simulink model "gm_HDLLDPCEncoder_vs"  (R2024a)
settings: Solver=FixedStepDiscrete  StartTime=0.0  StopTime=stopTime  RelTol=1e-3
values from neighbouring files (symbols this model uses):
  fs = 1    [testLDPCEncoder.m]
undefined symbols (not defined in the file or in its folder): clk, clk_enable, reset_x
libraries: whdlutilities x14, whdledac x6, simulink x5, dspsrcs4 x4, hdlsllib x1, vivadosimlib x1, HDL_ieee_8021513 x1
settings Model: Creator=cotti  LastModifiedBy=cotti
settings OptimizationCC: BlockReduction=off  ConditionallyExecuteInputs=off  DefaultParameterBehavior=Inlined  InheritOutputTypeSmallerThanSingle=on  ReuseModelBlockBuffer=off
settings DebuggingCC: AlgebraicLoopMsg=error  InheritedTsInSrcMsg=none  SingleTaskRateTransMsg=error  UnconnectedInputMsg=warning  UnconnectedOutputMsg=warning  UnconnectedLineMsg=warning
settings HardwareCC: ProdBitPerPointer=32  ProdBitPerSizeT=32  ProdBitPerPtrDiffT=32  ProdLargestAtomicFloat=None  ProdIntDivRoundTo=Undefined  ProdEndianess=Unspecified  ProdWordSize=32  ProdHWDeviceType=ASIC/FPGA->ASIC/FPGA  TargetBitPerLong=64  TargetBitPerPointer=64  TargetBitPerSizeT=64  TargetBitPerPtrDiffT=64  TargetLongLongMode=on  TargetIntDivRoundTo=Zero  TargetEndianess=LittleEndian  TargetWordSize=64  TargetHWDeviceType=Custom Processor->MATLAB Host Computer  ProdEqTarget=off
settings RTWCC: GPUComputeCapability=3.5

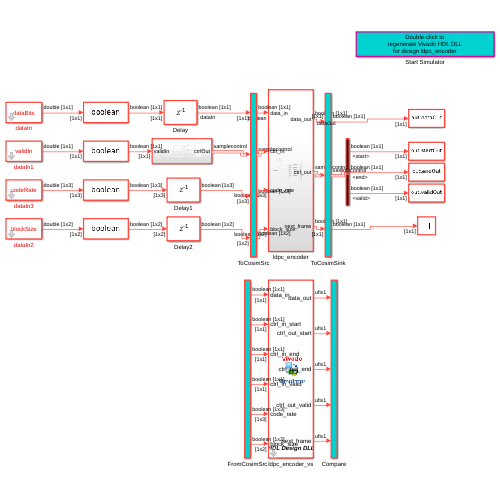
[thumbnail: Simulink's stored preview of the top-level diagram]
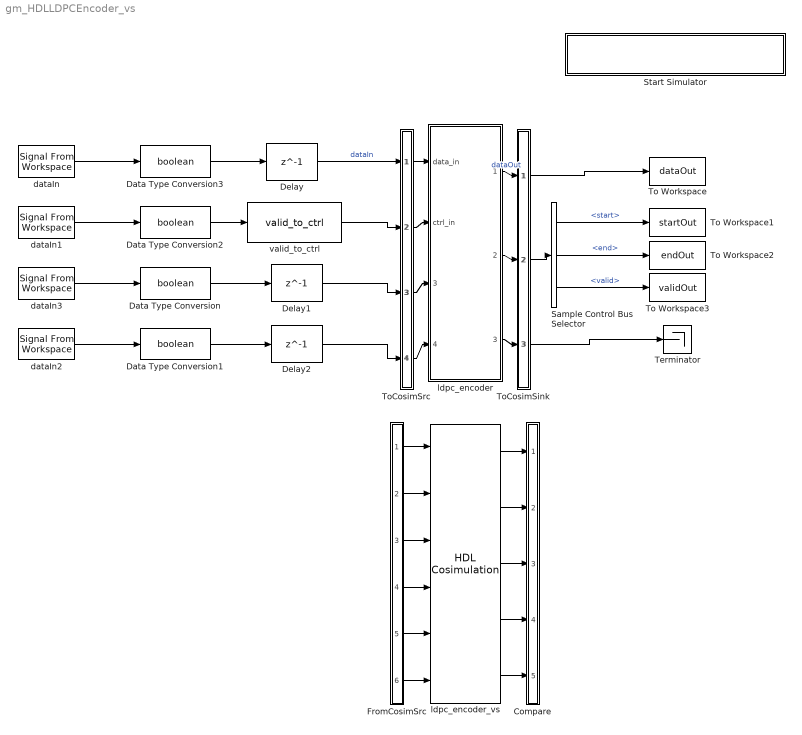
== system gm_HDLLDPCEncoder_vs ==
  Compare : Subsystem
      mask Display: disp('')
  Data Type Conversion{,1..3} (4 alike) : DataTypeConversion  OutDataTypeStr=boolean  SaturateOnIntegerOverflow=off  RndMeth=Floor
  Delay : Delay  DelayLength=1  InitialCondition=0  UseCircularBuffer=on
  Delay1 : Delay  DelayLength=1  InitialCondition=0  UseCircularBuffer=on
  Delay2 : Delay  DelayLength=1  InitialCondition=0  UseCircularBuffer=on
  FromCosimSrc : Subsystem
      mask Display: disp('')
  Sample Control Bus Selector : whdlutilities/Sample Control Bus Selector  OutputSignals=start,end,valid
  Start Simulator : Subsystem
      settings: OpenFcn=|
      | cosimDirName = pwd;
      | cd 'hdl_prj/hdlsrc/HDLLDPCEncoder';
      | [s,r] = system('vivado -mode batch -source gm_HDLLDPCEncoder_vs.tcl','-echo');
      | cd (cosimDirName);
      | clear cosimDirName;
      | if s
      |    error('Failed to create Vivado HDL design DLL using script gm_HDLLDPCEncoder_vs.tcl.');
      | end
      mask Display: disp('Double-click to\nregenerate Vivado HDL DLL\nfor design ldpc_encoder')
  Terminator : Terminator
  To Workspace : ToWorkspace  VariableName=dataOut  SampleTime=1/fs
      settings: Save2DSignal=2-D array (concatenate along first dimension)
  To Workspace1 : ToWorkspace  VariableName=startOut  SampleTime=1/fs
      settings: Save2DSignal=2-D array (concatenate along first dimension)
  To Workspace2 : ToWorkspace  VariableName=endOut  SampleTime=1/fs
      settings: Save2DSignal=2-D array (concatenate along first dimension)
  To Workspace3 : ToWorkspace  VariableName=validOut  SampleTime=1/fs
      settings: Save2DSignal=2-D array (concatenate along first dimension)
  ToCosimSink : Subsystem
      mask Display: disp('')
  ToCosimSrc : Subsystem
      mask Display: disp('')
  dataIn : dspsrcs4/Signal From Workspace  X=dataBits  Ts=1/fs  nsamps=1  OutputAfterFinalValue=Setting to zero  ignoreOrWarnInputAndFrameLengths=off  OutputFrames=off
  dataIn1 : dspsrcs4/Signal From Workspace  X=validIn  Ts=1/fs  nsamps=1  OutputAfterFinalValue=Setting to zero  ignoreOrWarnInputAndFrameLengths=off  OutputFrames=off
  dataIn2 : dspsrcs4/Signal From Workspace  X=blockSize  Ts=1/fs  nsamps=1  OutputAfterFinalValue=Setting to zero  ignoreOrWarnInputAndFrameLengths=off  OutputFrames=off
  dataIn3 : dspsrcs4/Signal From Workspace  X=codeRate  Ts=1/fs  nsamps=1  OutputAfterFinalValue=Setting to zero  ignoreOrWarnInputAndFrameLengths=off  OutputFrames=off
  ldpc_encoder : Subsystem
  ldpc_encoder_vs : vivadosimlib/HDL Cosimulation  PortPaths=/ldpc_encoder/data_in;/ldpc_encoder/ctrl_in_start;/ldpc_encoder/ctrl_in_end;/ldpc_encoder/ctrl_in_valid;/ldpc_encoder/code_rate;/ldpc_encoder/block_size;/ldpc_encoder/data_out;/ldpc_encoder/ctrl_out_start;/ldpc_encoder/ctrl_out_end;/ldpc_encoder/ctrl_out_valid;/ldpc_encoder/next_frame  PortModes=[1 1 1 1 1 1 2 2 2 2 2 ]  PortTimes=[-1 -1 -1 -1 -1 -1 1 1 1 1 1 ]  PortSigns=[-1 -1 -1 -1 -1 -1 0 0 0 0 0 ]  PortFracLengths=[0,0,0,0,0,0,0,0,0,0,0]  PortWordLengths=[-1,-1,-1,-1,-1,-1,1,1,1,1,1]  PortHDLWordSizes=[1,1,1,1,1,1,1,1,1,1,1]  CommLocal=on  CommSharedMemory=on  CommPortNumber=4449  CommShowInfo=on  ClockPaths=clk;clk_enable;reset_x;  ClockModes=[2 4 3]  ClockTimes=[1e-08 3.7e-08 2.7e-08]  TclPostSimCommand="puts \"done\""  TimingMode=ns  TimingScaleFactor=10  idxCellArray={'UNUSED_VAR'}  CosimBypass=Full Simulation  AllowDirectFeedthrough=on  ProductName=EDA Simulator Link VS  RunAutoTimescale=off  HdlClocks=0  PreRunTime=40  PreRunTimeUnit=ns
  valid_to_ctrl : HDL_ieee_8021513/valid_to_ctrl  SystemSampleTime=-1  VariantActivationTime=update diagram  AllowFlexibleInterface=on  Latency=0  AutoFrameSizeCalculation=off
      settings: SourceProductName=HDL IEEE 8021513
  wires:
  dataIn3/1 -> Data Type Conversion/1
  dataIn2/1 -> Data Type Conversion1/1
  dataIn/1 -> Data Type Conversion3/1
  Data Type Conversion/1 -> Delay1/1
  Data Type Conversion1/1 -> Delay2/1
  Data Type Conversion3/1 -> Delay/1
  dataIn1/1 -> Data Type Conversion2/1
  Data Type Conversion2/1 -> valid_to_ctrl/1
  Sample Control Bus Selector/3 -> To Workspace3/1  "<valid>"
  Sample Control Bus Selector/2 -> To Workspace2/1  "<end>"
  Sample Control Bus Selector/1 -> To Workspace1/1  "<start>"
  ToCosimSrc/1(out1) -> ldpc_encoder/1(data_in)
  ToCosimSrc/2(out2) -> ldpc_encoder/2(ctrl_in)
  ToCosimSrc/3(out3) -> ldpc_encoder/3(code_rate)
  ToCosimSrc/4(out4) -> ldpc_encoder/4(block_size)
  ldpc_encoder/1(data_out) -> ToCosimSink/1(in1)  "dataOut"
  ldpc_encoder/2(ctrl_out) -> ToCosimSink/2(in2)
  ldpc_encoder/3(next_frame) -> ToCosimSink/3(in3)
  Delay/1 -> ToCosimSrc/1(in1)  "dataIn"
  valid_to_ctrl/1 -> ToCosimSrc/2(in2)
  Delay1/1 -> ToCosimSrc/3(in3)
  Delay2/1 -> ToCosimSrc/4(in4)
  ToCosimSink/1(out1) -> To Workspace/1
  ToCosimSink/2(out2) -> Sample Control Bus Selector/1
  ToCosimSink/3(out3) -> Terminator/1
  FromCosimSrc/1(out1) -> ldpc_encoder_vs/1
  FromCosimSrc/2(out2) -> ldpc_encoder_vs/2
  FromCosimSrc/3(out3) -> ldpc_encoder_vs/3
  FromCosimSrc/4(out4) -> ldpc_encoder_vs/4
  FromCosimSrc/5(out5) -> ldpc_encoder_vs/5
  FromCosimSrc/6(out6) -> ldpc_encoder_vs/6
  ldpc_encoder_vs/1 -> Compare/1(in1)
  ldpc_encoder_vs/2 -> Compare/2(in2)
  ldpc_encoder_vs/3 -> Compare/3(in3)
  ldpc_encoder_vs/4 -> Compare/4(in4)
  ldpc_encoder_vs/5 -> Compare/5(in5)

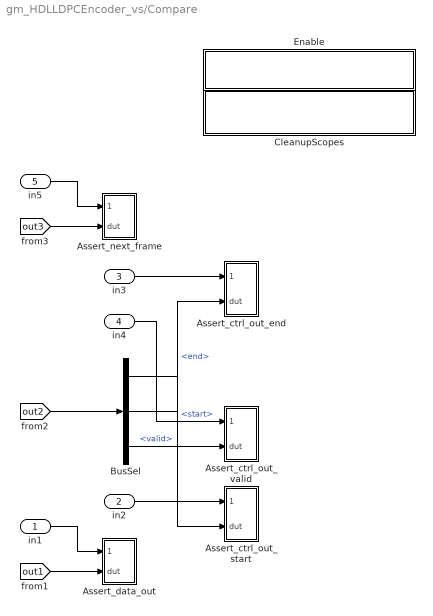
== system gm_HDLLDPCEncoder_vs/Compare ==
  in1 : Inport
  in2 : Inport  Port=2
  in3 : Inport  Port=3
  in4 : Inport  Port=4
  in5 : Inport  Port=5
  Assert_ctrl_out_end : Subsystem
      settings: LibrarySourceBlock=hdlmdlgenlib/AssertEq
  Assert_ctrl_out_start : Subsystem
      settings: LibrarySourceBlock=hdlmdlgenlib/AssertEq
  Assert_ctrl_out_valid : Subsystem
      settings: LibrarySourceBlock=hdlmdlgenlib/AssertEq
  Assert_data_out : Subsystem
      settings: LibrarySourceBlock=hdlmdlgenlib/AssertEq
  Assert_next_frame : Subsystem
      settings: LibrarySourceBlock=hdlmdlgenlib/AssertEq
  BusSel : BusSelector  OutputSignals=start,end,valid
  CleanupScopes : Subsystem
      settings: OpenFcn=|
      | blkName = gcb; %self block
      | idx = regexp(blkName, '/CleanupScopes$', 'once');
      | blkParent = blkName(1:idx-1);
      | blks=find_system(blkParent, 'LookUnderMasks', 'all','blocktype', 'Scope');
      | for itr = 1:length(blks)
      | 	 hScopeCfg = get_param(blks{itr},'ScopeConfiguration');
      | 	 hScopeCfg.Visible = ~ hScopeCfg.Visible;
      | end
      | drawnow;
      mask Display: fprintf(message('hdlcoder:cosim:vnl_dblclick').getString());
  Enable : Subsystem
      settings: OpenFcn=|
      | blkName = gcb;
      | idx = regexp(blkName, '/Enable$', 'once');
      | blkParent = blkName(1:idx-1);
      | blks=find_system(blkParent, 'LookUnderMasks', 'all','blocktype', 'Assertion');
      | e = get_param(blks{1}, 'Enabled');
      | if strcmp(e, 'on'), f= 'off';, else, f = 'on';, end
      | for ii=1:length(blks), set_param(blks{ii}, 'Enabled', f);, end
      | set_param(gcb, 'MaskDisplay',['fprintf(message(''hdlcoder:cosim:vnl_dblclick_assertions'',','''',upper(e),'''',').getString())']);
      mask Display: fprintf(message('hdlcoder:cosim:vnl_dblclick_assertions','OFF').getString());
  wires:
  in2/1 -> Assert_ctrl_out_start/1(cosim)
  BusSel/3 -> Assert_ctrl_out_valid/2(dut)  "<valid>"
  BusSel/2 -> Assert_ctrl_out_end/2(dut)  "<end>"
  in4/1 -> Assert_ctrl_out_valid/1(cosim)
  in3/1 -> Assert_ctrl_out_end/1(cosim)
  [out1] -> Assert_data_out/2(dut)
  [out2] -> BusSel/1
  BusSel/1 -> Assert_ctrl_out_start/2(dut)  "<start>"
  [out3] -> Assert_next_frame/2(dut)
  in1/1 -> Assert_data_out/1(cosim)
  in5/1 -> Assert_next_frame/1(cosim)

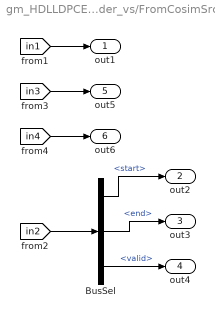
== system gm_HDLLDPCEncoder_vs/FromCosimSrc ==
  BusSel : BusSelector  OutputSignals=start,end,valid
  out1 : Outport
  out2 : Outport  Port=2
  out3 : Outport  Port=3
  out4 : Outport  Port=4
  out5 : Outport  Port=5
  out6 : Outport  Port=6
  wires:
  BusSel/3 -> out4/1  "<valid>"
  [in2] -> BusSel/1
  [in4] -> out6/1
  [in3] -> out5/1
  BusSel/2 -> out3/1  "<end>"
  BusSel/1 -> out2/1  "<start>"
  [in1] -> out1/1

== system gm_HDLLDPCEncoder_vs/Start Simulator ==

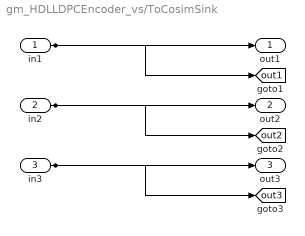
== system gm_HDLLDPCEncoder_vs/ToCosimSink ==
  in1 : Inport
  in2 : Inport  Port=2
  in3 : Inport  Port=3
  out1 : Outport
  out2 : Outport  Port=2
  out3 : Outport  Port=3
  tag scope: out1=global, out2=global, out3=global
  wires:
  in1/1 -> out1/1, [out1]
  in2/1 -> out2/1, [out2]
  in3/1 -> out3/1, [out3]

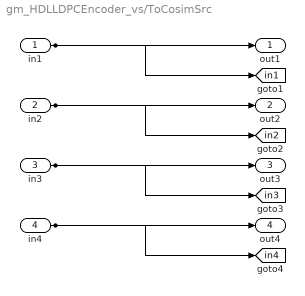
== system gm_HDLLDPCEncoder_vs/ToCosimSrc ==
  in1 : Inport
  in2 : Inport  Port=2
  in3 : Inport  Port=3
  in4 : Inport  Port=4
  out1 : Outport
  out2 : Outport  Port=2
  out3 : Outport  Port=3
  out4 : Outport  Port=4
  tag scope: in1=global, in2=global, in3=global, in4=global
  wires:
  in1/1 -> out1/1, [in1]
  in2/1 -> out2/1, [in2]
  in3/1 -> out3/1, [in3]
  in4/1 -> out4/1, [in4]

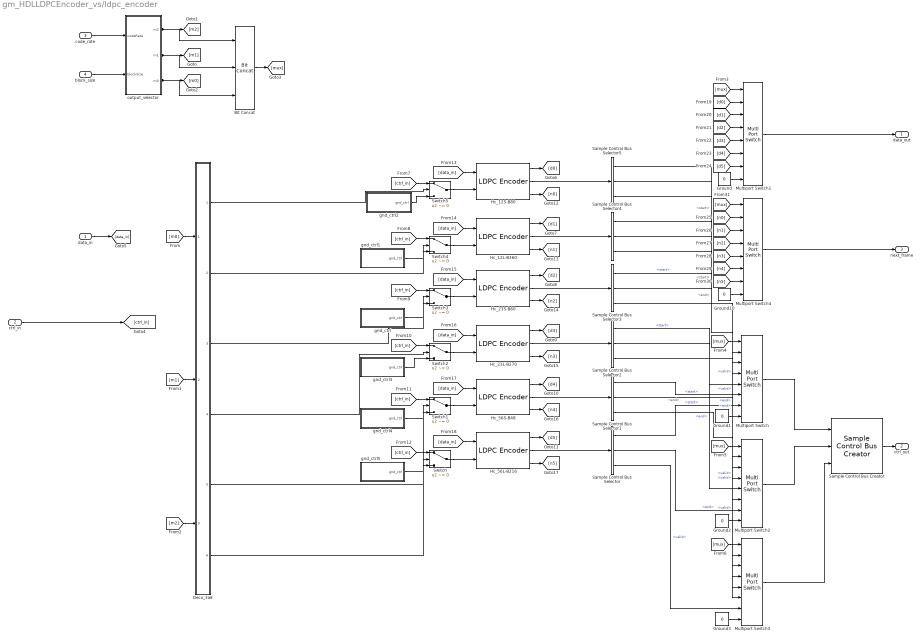
== system gm_HDLLDPCEncoder_vs/ldpc_encoder ==
  data_in : Inport  OutDataTypeStr=boolean  PortDimensions=1  SampleTime=1
  ctrl_in : Inport  Port=2
  code_rate : Inport  Port=3  OutDataTypeStr=boolean  PortDimensions=[1 3]  SampleTime=1
  block_size : Inport  Port=4  OutDataTypeStr=boolean  PortDimensions=[1 2]  SampleTime=1
  Bit Concat : hdlsllib/Logic and Bit Operations/Bit Concat  numInputs=3
  Deco_3a8 : Subsystem
  Ground{,1..3,10} (5 alike) : Constant  Value=0  OutDataTypeStr=boolean  SampleTime=-1
  Hc_12L-B360 : whdledac/LDPC Encoder  ParityCheckMatrix=Hc_12L  BlockSize=360  SimulateUsing=Code generation
  Hc_12S-B80 : whdledac/LDPC Encoder  ParityCheckMatrix=Hc_12S  BlockSize=80  SimulateUsing=Code generation
  Hc_23L-B270 : whdledac/LDPC Encoder  ParityCheckMatrix=Hc_23L  BlockSize=270  SimulateUsing=Code generation
  Hc_23S-B60 : whdledac/LDPC Encoder  ParityCheckMatrix=Hc_23S  BlockSize=60  SimulateUsing=Code generation
  Hc_56L-B216 : whdledac/LDPC Encoder  ParityCheckMatrix=Hc_56L  BlockSize=216  SimulateUsing=Code generation
  Hc_56S-B48 : whdledac/LDPC Encoder  ParityCheckMatrix=Hc_56S  BlockSize=48  SimulateUsing=Code generation
  Multiport Switch{,1..4} (5 alike) : MultiPortSwitch  DataPortOrder=Zero-based contiguous  Inputs=6  DataPortForDefault=Additional data port  DiagnosticForDefault=None  zeroidx=on  SaturateOnIntegerOverflow=off  InputSameDT=off
  Sample Control Bus Creator : whdlutilities/Sample Control Bus Creator
  Sample Control Bus Selector{,1..5} (6 alike) : whdlutilities/Sample Control Bus Selector  OutputSignals=start,end,valid
  Switch{,1..5} (6 alike) : Switch  Criteria=u2 ~= 0  SaturateOnIntegerOverflow=off  InputSameDT=off  OutDataTypeStr=Inherit: Same as first input
  gnd_ctrl : Subsystem
  gnd_ctrl1 : Subsystem
  gnd_ctrl2 : Subsystem
  gnd_ctrl3 : Subsystem
  gnd_ctrl4 : Subsystem
  gnd_ctrl5 : Subsystem
  output_selector : Subsystem
  data_out : Outport  SampleTime=1
  ctrl_out : Outport  Port=2
  next_frame : Outport  Port=3  SampleTime=1
  wires:
  output_selector/3(m0) -> [m0], Bit Concat/3
  output_selector/2(m1) -> [m1], Bit Concat/2
  output_selector/1(m2) -> [m2], Bit Concat/1
  gnd_ctrl5/1(gnd_ctrl) -> Switch/3
  gnd_ctrl4/1(gnd_ctrl) -> Switch1/3
  gnd_ctrl3/1(gnd_ctrl) -> Switch2/3
  gnd_ctrl2/1(gnd_ctrl) -> Switch5/3
  gnd_ctrl1/1(gnd_ctrl) -> Switch4/3
  gnd_ctrl/1(gnd_ctrl) -> Switch3/3
  Switch5/1 -> Hc_12S-B80/2
  Switch4/1 -> Hc_12L-B360/2
  Switch3/1 -> Hc_23S-B60/2
  Switch2/1 -> Hc_23L-B270/2
  Switch1/1 -> Hc_56S-B48/2
  Switch/1 -> Hc_56L-B216/2
  Sample Control Bus Selector5/3 -> Multiport Switch3/2  "<valid>"
  Sample Control Bus Selector5/2 -> Multiport Switch2/2  "<end>"
  Sample Control Bus Selector5/1 -> Multiport Switch/2  "<start>"
  Sample Control Bus Selector4/3 -> Multiport Switch3/3  "<valid>"
  Sample Control Bus Selector4/2 -> Multiport Switch2/3  "<end>"
  Sample Control Bus Selector4/1 -> Multiport Switch/3  "<start>"
  Sample Control Bus Selector3/3 -> Multiport Switch3/4  "<valid>"
  Sample Control Bus Selector3/2 -> Multiport Switch2/4  "<end>"
  Sample Control Bus Selector3/1 -> Multiport Switch/4  "<start>"
  Sample Control Bus Selector2/3 -> Multiport Switch3/5  "<valid>"
  Sample Control Bus Selector2/2 -> Multiport Switch2/5  "<end>"
  Sample Control Bus Selector2/1 -> Multiport Switch/5  "<start>"
  Sample Control Bus Selector1/3 -> Multiport Switch3/6  "<valid>"
  Sample Control Bus Selector1/2 -> Multiport Switch2/6  "<end>"
  Sample Control Bus Selector1/1 -> Multiport Switch/6  "<start>"
  Sample Control Bus Selector/3 -> Multiport Switch3/7  "<valid>"
  Sample Control Bus Selector/2 -> Multiport Switch2/7  "<end>"
  Sample Control Bus Selector/1 -> Multiport Switch/7  "<start>"
  Sample Control Bus Creator/1 -> ctrl_out/1
  Multiport Switch4/1 -> next_frame/1
  Multiport Switch3/1 -> Sample Control Bus Creator/3
  Multiport Switch2/1 -> Sample Control Bus Creator/2
  Multiport Switch1/1 -> data_out/1
  Multiport Switch/1 -> Sample Control Bus Creator/1
  Hc_56S-B48/3 -> [n4]
  Hc_56S-B48/2 -> Sample Control Bus Selector1/1
  Hc_56S-B48/1 -> [d4]
  Hc_56L-B216/3 -> [n5]
  Hc_56L-B216/2 -> Sample Control Bus Selector/1
  Hc_56L-B216/1 -> [d5]
  Hc_23S-B60/3 -> [n2]
  Hc_23S-B60/2 -> Sample Control Bus Selector3/1
  Hc_23S-B60/1 -> [d2]
  Hc_23L-B270/3 -> [n3]
  Hc_23L-B270/2 -> Sample Control Bus Selector2/1
  Hc_23L-B270/1 -> [d3]
  Hc_12S-B80/3 -> [n0]
  Hc_12S-B80/2 -> Sample Control Bus Selector5/1
  Hc_12S-B80/1 -> [d0]
  Hc_12L-B360/3 -> [n1]
  Hc_12L-B360/2 -> Sample Control Bus Selector4/1
  Hc_12L-B360/1 -> [d1]
  Ground3/1 -> Multiport Switch3/8
  Ground2/1 -> Multiport Switch2/8
  Ground10/1 -> Multiport Switch4/8
  Ground1/1 -> Multiport Switch/8
  Ground/1 -> Multiport Switch1/8
  [ctrl_in] -> Switch3/1
  [ctrl_in] -> Switch4/1
  [ctrl_in] -> Switch5/1
  [mux] -> Multiport Switch3/1
  [mux] -> Multiport Switch2/1
  [mux] -> Multiport Switch/1
  [mux] -> Multiport Switch4/1
  [n5] -> Multiport Switch4/7
  [mux] -> Multiport Switch1/1
  [n4] -> Multiport Switch4/6
  [n3] -> Multiport Switch4/5
  [n2] -> Multiport Switch4/4
  [n1] -> Multiport Switch4/3
  [n0] -> Multiport Switch4/2
  [d5] -> Multiport Switch1/7
  [d4] -> Multiport Switch1/6
  [d3] -> Multiport Switch1/5
  [d2] -> Multiport Switch1/4
  [d1] -> Multiport Switch1/3
  [m2] -> Deco_3a8/3(in2)
  [d0] -> Multiport Switch1/2
  [data_in] -> Hc_56L-B216/1
  [data_in] -> Hc_56S-B48/1
  [data_in] -> Hc_23L-B270/1
  [data_in] -> Hc_23S-B60/1
  [data_in] -> Hc_12L-B360/1
  [data_in] -> Hc_12S-B80/1
  [ctrl_in] -> Switch/1
  [ctrl_in] -> Switch1/1
  [ctrl_in] -> Switch2/1
  [m1] -> Deco_3a8/2(in1)
  [m0] -> Deco_3a8/1(in0)
  Deco_3a8/6(m5) -> Switch/2
  Deco_3a8/5(m4) -> Switch1/2
  Deco_3a8/4(m3) -> Switch2/2
  Deco_3a8/3(m2) -> Switch3/2
  Deco_3a8/2(m1) -> Switch4/2
  Deco_3a8/1(m0) -> Switch5/2
  Bit Concat/1 -> [mux]
  block_size/1 -> output_selector/2(blockSize)
  code_rate/1 -> output_selector/1(codeRate)
  ctrl_in/1 -> [ctrl_in]
  data_in/1 -> [data_in]

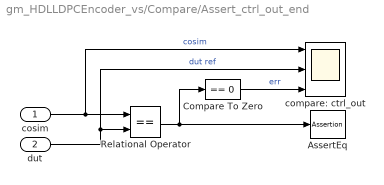
== system gm_HDLLDPCEncoder_vs/Compare/Assert_ctrl_out_end ==
  cosim : Inport
  dut : Inport  Port=2
  AssertEq : Assertion
  Compare To Zero : simulink/Logic and Bit Operations/Compare To Zero  relop===  OutDataTypeStr=boolean
  Relational Operator : RelationalOperator  Operator===  OutDataTypeStr=boolean  InputSameDT=off
  compare: ctrl_out : Scope  NumInputPorts=3
  wires:
  Compare To Zero/1 -> compare: ctrl_out/3  "err"
  Relational Operator/1 -> Compare To Zero/1, AssertEq/1
  cosim/1 -> compare: ctrl_out/1, Relational Operator/1  "cosim"
  dut/1 -> compare: ctrl_out/2, Relational Operator/2  "dut ref"

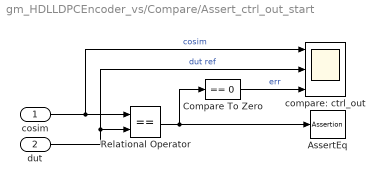
== system gm_HDLLDPCEncoder_vs/Compare/Assert_ctrl_out_start ==
  cosim : Inport
  dut : Inport  Port=2
  AssertEq : Assertion
  Compare To Zero : simulink/Logic and Bit Operations/Compare To Zero  relop===  OutDataTypeStr=boolean
  Relational Operator : RelationalOperator  Operator===  OutDataTypeStr=boolean  InputSameDT=off
  compare: ctrl_out : Scope  NumInputPorts=3
  wires:
  Compare To Zero/1 -> compare: ctrl_out/3  "err"
  Relational Operator/1 -> Compare To Zero/1, AssertEq/1
  cosim/1 -> compare: ctrl_out/1, Relational Operator/1  "cosim"
  dut/1 -> compare: ctrl_out/2, Relational Operator/2  "dut ref"

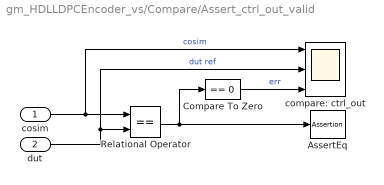
== system gm_HDLLDPCEncoder_vs/Compare/Assert_ctrl_out_valid ==
  cosim : Inport
  dut : Inport  Port=2
  AssertEq : Assertion
  Compare To Zero : simulink/Logic and Bit Operations/Compare To Zero  relop===  OutDataTypeStr=boolean
  Relational Operator : RelationalOperator  Operator===  OutDataTypeStr=boolean  InputSameDT=off
  compare: ctrl_out : Scope  NumInputPorts=3
  wires:
  Compare To Zero/1 -> compare: ctrl_out/3  "err"
  Relational Operator/1 -> Compare To Zero/1, AssertEq/1
  cosim/1 -> compare: ctrl_out/1, Relational Operator/1  "cosim"
  dut/1 -> compare: ctrl_out/2, Relational Operator/2  "dut ref"

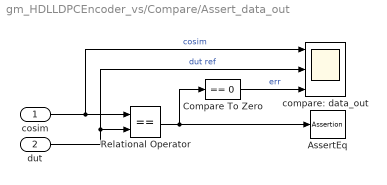
== system gm_HDLLDPCEncoder_vs/Compare/Assert_data_out ==
  cosim : Inport
  dut : Inport  Port=2
  AssertEq : Assertion
  Compare To Zero : simulink/Logic and Bit Operations/Compare To Zero  relop===  OutDataTypeStr=boolean
  Relational Operator : RelationalOperator  Operator===  OutDataTypeStr=boolean  InputSameDT=off
  compare: data_out : Scope  NumInputPorts=3
  wires:
  Compare To Zero/1 -> compare: data_out/3  "err"
  Relational Operator/1 -> Compare To Zero/1, AssertEq/1
  cosim/1 -> compare: data_out/1, Relational Operator/1  "cosim"
  dut/1 -> compare: data_out/2, Relational Operator/2  "dut ref"

== system gm_HDLLDPCEncoder_vs/Compare/Assert_next_frame ==
  cosim : Inport
  dut : Inport  Port=2
  AssertEq : Assertion
  Compare To Zero : simulink/Logic and Bit Operations/Compare To Zero  relop===  OutDataTypeStr=boolean
  Relational Operator : RelationalOperator  Operator===  OutDataTypeStr=boolean  InputSameDT=off
  compare: next_frame : Scope  NumInputPorts=3
  wires:
  Compare To Zero/1 -> compare: next_frame/3  "err"
  Relational Operator/1 -> Compare To Zero/1, AssertEq/1
  cosim/1 -> compare: next_frame/1, Relational Operator/1  "cosim"
  dut/1 -> compare: next_frame/2, Relational Operator/2  "dut ref"

== system gm_HDLLDPCEncoder_vs/Compare/CleanupScopes ==

== system gm_HDLLDPCEncoder_vs/Compare/Enable ==

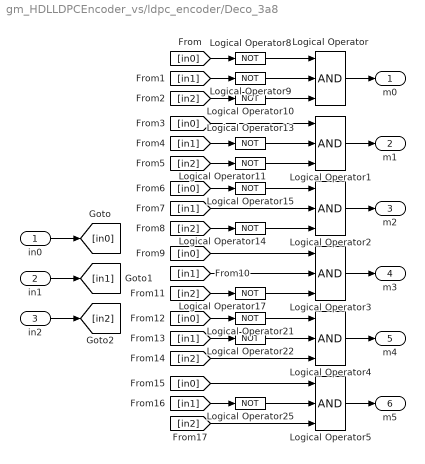
== system gm_HDLLDPCEncoder_vs/ldpc_encoder/Deco_3a8 ==
  in0 : Inport  OutDataTypeStr=boolean  SampleTime=1
  in1 : Inport  Port=2  OutDataTypeStr=boolean  SampleTime=1
  in2 : Inport  Port=3  OutDataTypeStr=boolean  SampleTime=1
  Logical Operator{,1..5} (6 alike) : Logic  Inputs=3  IconShape=distinctive  AllPortsSameDT=off  OutDataTypeStr=boolean
  Logical Operator{8..11,13..15,17,21..22,25} (11 alike) : Logic  Operator=NOT  IconShape=distinctive  AllPortsSameDT=off  OutDataTypeStr=boolean
  m0 : Outport  SampleTime=1
  m1 : Outport  Port=2  SampleTime=1
  m2 : Outport  Port=3  SampleTime=1
  m3 : Outport  Port=4  SampleTime=1
  m4 : Outport  Port=5  SampleTime=1
  m5 : Outport  Port=6  SampleTime=1
  wires:
  Logical Operator9/1 -> Logical Operator/2
  Logical Operator8/1 -> Logical Operator/1
  Logical Operator5/1 -> m5/1
  Logical Operator4/1 -> m4/1
  Logical Operator3/1 -> m3/1
  Logical Operator25/1 -> Logical Operator5/2
  Logical Operator22/1 -> Logical Operator4/2
  Logical Operator21/1 -> Logical Operator4/1
  Logical Operator2/1 -> m2/1
  Logical Operator17/1 -> Logical Operator3/3
  Logical Operator15/1 -> Logical Operator2/1
  Logical Operator14/1 -> Logical Operator2/3
  Logical Operator13/1 -> Logical Operator1/2
  Logical Operator11/1 -> Logical Operator1/3
  Logical Operator10/1 -> Logical Operator/3
  Logical Operator1/1 -> m1/1
  Logical Operator/1 -> m0/1
  [in0] -> Logical Operator3/1
  [in2] -> Logical Operator14/1
  [in1] -> Logical Operator2/2
  [in0] -> Logical Operator15/1
  [in2] -> Logical Operator11/1
  [in1] -> Logical Operator13/1
  [in0] -> Logical Operator1/1
  [in2] -> Logical Operator10/1
  [in2] -> Logical Operator5/3
  [in1] -> Logical Operator25/1
  [in0] -> Logical Operator5/1
  [in2] -> Logical Operator4/3
  [in1] -> Logical Operator22/1
  [in0] -> Logical Operator21/1
  [in2] -> Logical Operator17/1
  [in1] -> Logical Operator3/2
  [in1] -> Logical Operator9/1
  [in0] -> Logical Operator8/1
  in2/1 -> [in2]
  in1/1 -> [in1]
  in0/1 -> [in0]

== system gm_HDLLDPCEncoder_vs/ldpc_encoder/gnd_ctrl ==
  Ground : Ground
  Ground1 : Ground
  Ground2 : Ground
  Sample Control Bus Creator : whdlutilities/Sample Control Bus Creator
  gnd_ctrl : Outport  SampleTime=1
  wires:
  Sample Control Bus Creator/1 -> gnd_ctrl/1
  Ground2/1 -> Sample Control Bus Creator/1
  Ground1/1 -> Sample Control Bus Creator/2
  Ground/1 -> Sample Control Bus Creator/3

== system gm_HDLLDPCEncoder_vs/ldpc_encoder/gnd_ctrl1 ==
  Ground : Ground
  Ground1 : Ground
  Ground2 : Ground
  Sample Control Bus Creator : whdlutilities/Sample Control Bus Creator
  gnd_ctrl : Outport  SampleTime=1
  wires:
  Sample Control Bus Creator/1 -> gnd_ctrl/1
  Ground2/1 -> Sample Control Bus Creator/1
  Ground1/1 -> Sample Control Bus Creator/2
  Ground/1 -> Sample Control Bus Creator/3

== system gm_HDLLDPCEncoder_vs/ldpc_encoder/gnd_ctrl2 ==
  Ground : Ground
  Ground1 : Ground
  Ground2 : Ground
  Sample Control Bus Creator : whdlutilities/Sample Control Bus Creator
  gnd_ctrl : Outport  SampleTime=1
  wires:
  Sample Control Bus Creator/1 -> gnd_ctrl/1
  Ground2/1 -> Sample Control Bus Creator/1
  Ground1/1 -> Sample Control Bus Creator/2
  Ground/1 -> Sample Control Bus Creator/3

== system gm_HDLLDPCEncoder_vs/ldpc_encoder/gnd_ctrl3 ==
  Ground : Ground
  Ground1 : Ground
  Ground2 : Ground
  Sample Control Bus Creator : whdlutilities/Sample Control Bus Creator
  gnd_ctrl : Outport  SampleTime=1
  wires:
  Sample Control Bus Creator/1 -> gnd_ctrl/1
  Ground2/1 -> Sample Control Bus Creator/1
  Ground1/1 -> Sample Control Bus Creator/2
  Ground/1 -> Sample Control Bus Creator/3

== system gm_HDLLDPCEncoder_vs/ldpc_encoder/gnd_ctrl4 ==
  Ground : Ground
  Ground1 : Ground
  Ground2 : Ground
  Sample Control Bus Creator : whdlutilities/Sample Control Bus Creator
  gnd_ctrl : Outport  SampleTime=1
  wires:
  Sample Control Bus Creator/1 -> gnd_ctrl/1
  Ground2/1 -> Sample Control Bus Creator/1
  Ground1/1 -> Sample Control Bus Creator/2
  Ground/1 -> Sample Control Bus Creator/3

== system gm_HDLLDPCEncoder_vs/ldpc_encoder/gnd_ctrl5 ==
  Ground : Ground
  Ground1 : Ground
  Ground2 : Ground
  Sample Control Bus Creator : whdlutilities/Sample Control Bus Creator
  gnd_ctrl : Outport  SampleTime=1
  wires:
  Sample Control Bus Creator/1 -> gnd_ctrl/1
  Ground2/1 -> Sample Control Bus Creator/1
  Ground1/1 -> Sample Control Bus Creator/2
  Ground/1 -> Sample Control Bus Creator/3

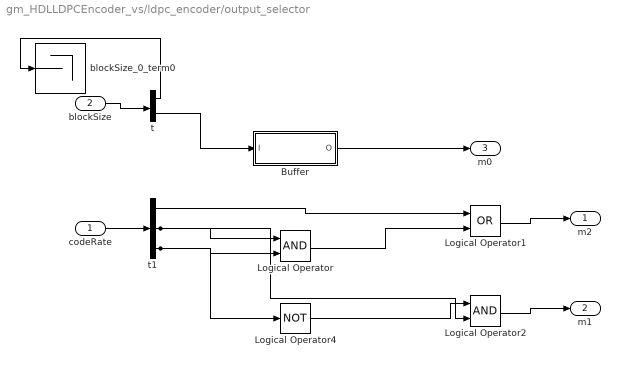
== system gm_HDLLDPCEncoder_vs/ldpc_encoder/output_selector ==
  codeRate : Inport  OutDataTypeStr=boolean  PortDimensions=[1 3]  SampleTime=1
  blockSize : Inport  Port=2  OutDataTypeStr=boolean  PortDimensions=[1 2]  SampleTime=1
  Buffer : Subsystem
  Logical Operator : Logic  AllPortsSameDT=off  OutDataTypeStr=boolean  SampleTime=1
  Logical Operator1 : Logic  Operator=OR  AllPortsSameDT=off  OutDataTypeStr=boolean  SampleTime=1
  Logical Operator2 : Logic  AllPortsSameDT=off  OutDataTypeStr=boolean  SampleTime=1
  Logical Operator4 : Logic  Operator=NOT  Inputs=1  AllPortsSameDT=off  OutDataTypeStr=boolean  SampleTime=1
  blockSize_0_term0 : Terminator
  t : Demux  Outputs=2
  t1 : Demux  Outputs=3
  m2 : Outport  SampleTime=1  VectorParamsAs1DForOutWhenUnconnected=off
  m1 : Outport  Port=2  SampleTime=1  VectorParamsAs1DForOutWhenUnconnected=off
  m0 : Outport  Port=3  SampleTime=1  VectorParamsAs1DForOutWhenUnconnected=off
  wires:
  t/1 -> blockSize_0_term0/1
  Logical Operator4/1 -> Logical Operator2/1
  Logical Operator2/1 -> m1/1
  Logical Operator1/1 -> m2/1
  Logical Operator/1 -> Logical Operator1/2
  t1/3 -> Logical Operator/2, Logical Operator4/1
  t1/2 -> Logical Operator/1, Logical Operator2/2
  t1/1 -> Logical Operator1/1
  t/2 -> Buffer/1(I)
  Buffer/1(O) -> m0/1
  blockSize/1 -> t/1
  codeRate/1 -> t1/1

== system gm_HDLLDPCEncoder_vs/ldpc_encoder/output_selector/Buffer ==
  I : Inport  OutDataTypeStr=boolean  SampleTime=1
  O : Outport  SampleTime=1
  wires:
  I/1 -> O/1
